simulink model "sedemo_triggergate_v_valuechangegate"  (Simulink 7.5)
settings: Solver=VariableStepDiscrete  StartTime=0.0  StopTime=10.0  MaxStep=inf  RelTol=1e-3
libraries: simeventssink1 x3, simeventsqueue1 x2, simeventsgates1 x2, simeventsgenerators1 x2, simulink x1
settings Model: Creator=The MathWorks Inc.  ExtModeAutoUpdateStatusClock=off
settings DataIOCC: SaveOutput=off  SaveTime=off
settings OptimizationCC: InitFltsAndDblsToZero=on
settings DebuggingCC: AlgebraicLoopMsg=error  SaveWithParameterizedLinksMsg=none  SignalResolutionControl=TryResolveAllWithWarning  SolverPrmCheckMsg=none  MultiTaskDSMMsg=warning  MultiTaskCondExecSysMsg=none  SigSpecEnsureSampleTimeMsg=none  StrictBusMsg=None
settings RTWCC: IncludeERTFirstTime=on
settings GRTTargetCC: TargetFcnLib=ansi_tfl_tmw.mat
settings SimEventsCC: propIdentEventSeed=12345678  propDiagAttribOutput=1  propDiagFcnCallOutput=1  propDiagStatOutput=0

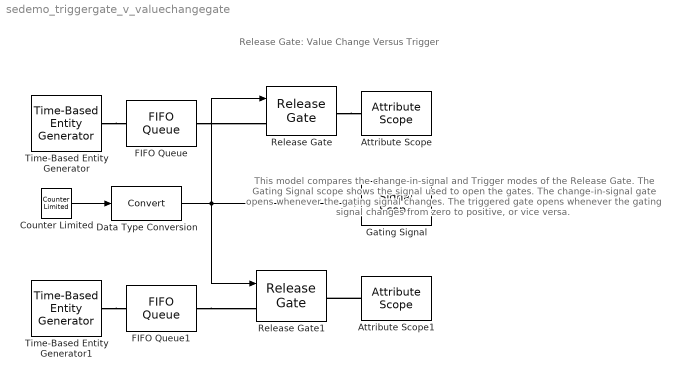
== system sedemo_triggergate_v_valuechangegate ==
  note: Release Gate: Value Change Versus Trigger
  note: This model compares the
      | change-in-signal and Trigger modes
      | of the Release Gate.
      |
      | The Gating Signal scope shows the
      | signal used to open the gates.
      |
      | The change-in-signal gate opens
      | whenever the gating signal changes.
      |
      | The triggered gate opens whenever
      | the gating signal changes from zero
      | to positive, or vice versa.
  Attribute Scope : simeventssink1/Attribute Scope  Priority=1  SystemSampleTime=-1  PlotType=Stair  InputType=Attribute  NumInputs=1  AttributeNameY=Count  XInputOptionSignal=Event time  XInputOptionEntity=Event time  AttributeNameX=Count  EnableEntityOutport=off  XMin=0  XMax=10  XLimitExceededOption=Stretch axis limits  YLimitExceededOption=Stretch axis limits  AxisGrid=off  AxisLegend=off  LineDisables=""  LineColors=b  LineStyles=-  LineMarkers=x  OpenScopeAtSimStart=on  Title=Entities passing through Change-in-signal release gate  YLabel=""  XLabel=Time  FigurePosition=[685 548 334 150]  AxisZoom=off  DataStoreOption=Limited  DataPointsLimit=10000  StatNumberArrived=Off  ShowCountPlotted=off  ShowToolbar=on
      settings: YMin=-0.5  YMax=0.5
  Attribute Scope1 : simeventssink1/Attribute Scope  Priority=1  SystemSampleTime=-1  PlotType=Stair  InputType=Attribute  NumInputs=1  AttributeNameY=Count  XInputOptionSignal=Event time  XInputOptionEntity=Event time  AttributeNameX=Count  EnableEntityOutport=off  XMin=0  XMax=10  XLimitExceededOption=Stretch axis limits  YLimitExceededOption=Stretch axis limits  AxisGrid=off  AxisLegend=off  LineDisables=""  LineColors=b  LineStyles=-  LineMarkers=x  OpenScopeAtSimStart=on  Title=Entities passing through Trigger release gate  YLabel=""  XLabel=Time  FigurePosition=[685 100 334 149]  AxisZoom=off  DataStoreOption=Limited  DataPointsLimit=10000  StatNumberArrived=Off  ShowCountPlotted=off  ShowToolbar=on
      settings: YMin=-0.5  YMax=0.5
  Counter Limited : simulink/Sources/Counter Limited  SystemSampleTime=-1  uplimit=3  tsamp=0.5
  Data Type Conversion : DataTypeConversion  OutDataType=sfix(16)  OutScaling=2^0
  FIFO Queue : simeventsqueue1/FIFO Queue  Priority=1  SystemSampleTime=-1  Capacity=25  EnableTOPort=off  StatNumberDeparted=Off  StatNumberInBlock=Off  StatPendingEntity=Off  StatAverageWait=Off  StatAverageQueueLength=Off  StatNumberTimedout=Off
  FIFO Queue1 : simeventsqueue1/FIFO Queue  Priority=1  SystemSampleTime=-1  Capacity=25  EnableTOPort=off  StatNumberDeparted=Off  StatNumberInBlock=Off  StatPendingEntity=Off  StatAverageWait=Off  StatAverageQueueLength=Off  StatNumberTimedout=Off
  "Gating Signal " : simeventssink1/Signal Scope  Priority=1  SystemSampleTime=-1  PlotType=Stair  InputType=Signal  NumInputs=1  AttributeNameY=Count  XInputOptionSignal=Event time  XInputOptionEntity=Event time  AttributeNameX=Count  EnableEntityOutport=on  XMin=0  XMax=10  XLimitExceededOption=Stretch axis limits  YLimitExceededOption=Stretch axis limits  AxisGrid=on  AxisLegend=off  LineDisables=""  LineColors=b  LineStyles=-  LineMarkers=.  OpenScopeAtSimStart=on  Title=Gating Signal  YLabel=""  XLabel=Time  FigurePosition=[685 324 334 150]  AxisZoom=off  DataStoreOption=Limited  DataPointsLimit=10000  StatNumberArrived=Off  ShowCountPlotted=off  ShowToolbar=on
      settings: YMin=-0.5  YMax=3.5
  Release Gate : simeventsgates1/Release Gate  Priority=1  SystemSampleTime=-1  OpenGateUpon=Change in signal from port vc  SignalEdgeOption=Either  SpecifyEventPriority=on  PriorityGateRelease=2200  StatNumberDeparted=Off
      settings: AttributesFormatString=Open Gate on = %<OpenGateUpon>\nChange type = %<SignalEdgeOption>
  Release Gate1 : simeventsgates1/Release Gate  Priority=1  SystemSampleTime=-1  OpenGateUpon=Trigger from port tr  SignalEdgeOption=Either  SpecifyEventPriority=on  PriorityGateRelease=2200  StatNumberDeparted=Off
      settings: AttributesFormatString=Open Gate on = %<OpenGateUpon>\nChange type = %<SignalEdgeOption>
  Time-Based Entity Generator : simeventsgenerators1/Entity Generators/Time-Based Entity Generator  Priority=1  DialogController=des_ddg_create  DialogControllerArgs=DataTag8  SystemSampleTime=-1  GenerateEntitiesUpon=Intergeneration time from dialog  Distribution=Constant  Minimum=0  Maximum=1  Mean=1  InitialSeed=12345  Period=0.5  PriorityEntityGeneration=5000  GenerateEntityAtSimulationStart=on  ResponseWhenBlocked=Pause generation  ResponseWhenUnblocked=Immediate restart  EntityType=Standard  StatNumberDeparted=Off  StatPendingEntity=Off  StatAverageIntergenerationTime=Off
  Time-Based Entity Generator1 : simeventsgenerators1/Entity Generators/Time-Based Entity Generator  Priority=1  DialogController=des_ddg_create  DialogControllerArgs=DataTag10  SystemSampleTime=-1  GenerateEntitiesUpon=Intergeneration time from dialog  Distribution=Constant  Minimum=0  Maximum=1  Mean=1  InitialSeed=12345  Period=0.5  PriorityEntityGeneration=6000  GenerateEntityAtSimulationStart=on  ResponseWhenBlocked=Pause generation  ResponseWhenUnblocked=Immediate restart  EntityType=Standard  StatNumberDeparted=Off  StatPendingEntity=Off  StatAverageIntergenerationTime=Off
  wires:
  Counter Limited/1 -> Data Type Conversion/1
  Data Type Conversion/1 -> "Gating Signal "/1, Release Gate/1, Release Gate1/1
  connections:
  FIFO Queue/RConn1 -- Release Gate/LConn1
  FIFO Queue1/RConn1 -- Release Gate1/LConn1
  Release Gate/RConn1 -- Attribute Scope/LConn1
  Attribute Scope1/LConn1 -- Release Gate1/RConn1
  Time-Based Entity Generator/RConn1 -- FIFO Queue/LConn1
  Time-Based Entity Generator1/RConn1 -- FIFO Queue1/LConn1
